simulink model "LIMP"  (R2014b)
settings: Solver=ode3  StartTime=0.0  StopTime=10.0  FixedStep=0.01  RelTol=1e-3
values from neighbouring files (symbols this model uses):
  G = 9.81    [main.m]
  i = max(find(p > availablepercentiles))    [cmaes.m]
  x = 100 * (x.^2 - y) + (x - 1).^2    [cmaes.m]    (also in ddp_naive.m = zeros(nx, n+1); main.m = 0; p1_plan001.mat = [0 2.16226505425e-05 9.59496359766e-05 0.00022595251555 0.00; p1_sim.m = S(:, 1))
  xd = 0    [main.m]    (also in p1_plan001.mat = [0 0.000462576080308 0.00102632112351 0.0015734075806 0.0021; p1_sim.m = S(:, 3); processData.m = Sxd.Data(end))
  y = repmat(scale, 1, size(x,2)) .* x    [cmaes.m]    (also in main.m = 0; p1_plan001.mat = [0 -1.26027772298e-05 -5.49591014786e-05 -0.00012654563427 -; p1_sim.m = S(:, 2); p2_ddp_run.m = vars.y)
  yd = 0    [main.m]    (also in p1_plan001.mat = [0 -0.000268095565629 -0.000576196670308 -0.000853920776779 ; p1_sim.m = S(:, 4); processData.m = Syd.Data(end))
  z = 1    [main.m]
undefined symbols (not defined in the file or in its folder): limp
libraries: simulink x1
settings Model: Creator=tianyuchen  LastModifiedBy=tianyuchen

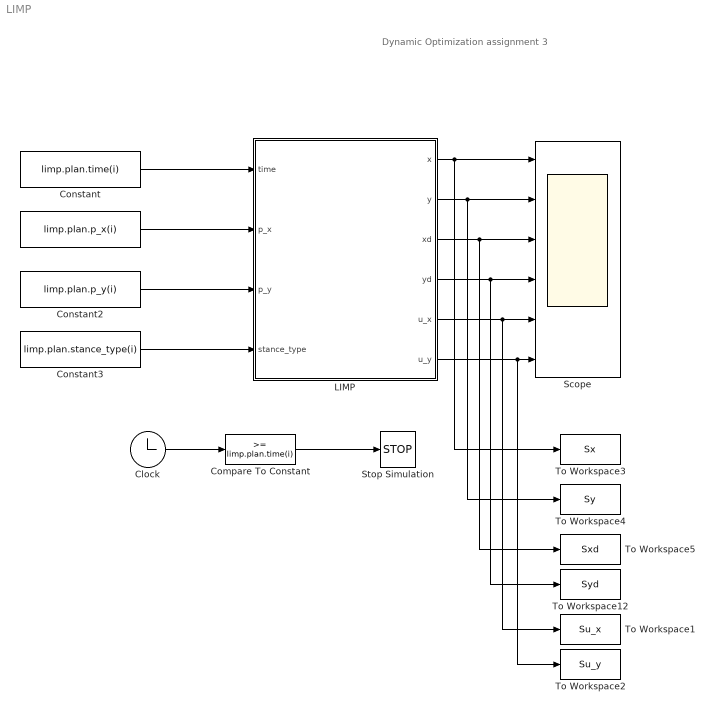
== system LIMP ==
  note: Dynamic Optimization
      | assignment 3
  " " : Constant  Value=limp.plan.p_x(i)
  Clock : Clock
  Compare To Constant : simulink/Logic and Bit Operations/Compare To Constant  relop=>=  const=limp.plan.time(i)  OutDataTypeStr=boolean
  Constant : Constant  Value=limp.plan.time(i)
  Constant2 : Constant  Value=limp.plan.p_y(i)
  Constant3 : Constant  Value=limp.plan.stance_type(i)
  LIMP : Subsystem
  Scope : Scope  NumInputPorts=6
      settings: TickLabels=on  ShowLegends=on  YMin=-5~-5~-5~-5~-5~-5  YMax=5~5~5~5~5~5  ScrollMode=on
  Stop Simulation : Stop
  To Workspace1 : ToWorkspace  VariableName=Su_x  SaveFormat=Timeseries  SampleTime=-1
  To Workspace12 : ToWorkspace  VariableName=Syd  SaveFormat=Timeseries  SampleTime=-1
  To Workspace2 : ToWorkspace  VariableName=Su_y  SaveFormat=Timeseries  SampleTime=-1
  To Workspace3 : ToWorkspace  VariableName=Sx  SaveFormat=Timeseries  SampleTime=-1
  To Workspace4 : ToWorkspace  VariableName=Sy  SaveFormat=Timeseries  SampleTime=-1
  To Workspace5 : ToWorkspace  VariableName=Sxd  SaveFormat=Timeseries  SampleTime=-1
  wires:
  Constant/1 -> LIMP/1(time)
  " "/1 -> LIMP/2(p_x)
  Constant2/1 -> LIMP/3(p_y)
  Constant3/1 -> LIMP/4(stance_type)
  Clock/1 -> Compare To Constant/1
  Compare To Constant/1 -> Stop Simulation/1
  LIMP/2(y) -> To Workspace4/1, Scope/2
  LIMP/3(xd) -> To Workspace5/1, Scope/3
  LIMP/4(yd) -> To Workspace12/1, Scope/4
  LIMP/6(u_y) -> To Workspace2/1, Scope/6
  LIMP/5(u_x) -> To Workspace1/1, Scope/5
  LIMP/1(x) -> To Workspace3/1, Scope/1

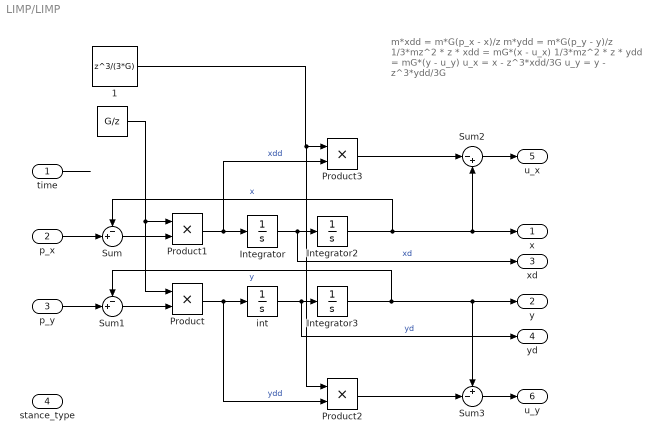
== system LIMP/LIMP ==
  note: m*xdd = m*G(p_x - x)/z
      | m*ydd = m*G(p_y - y)/z
      | 1/3*mz^2 * z * xdd = mG*(x - u_x)
      | 1/3*mz^2 * z * ydd = mG*(y - u_y)
      |
      | u_x = x - z^3*xdd/3G
      | u_y = y - z^3*ydd/3G
  time : Inport
  p_x : Inport  Port=2
  p_y : Inport  Port=3
  stance_type : Inport  Port=4
  " " : Constant  Value=G/z
  " 1" : Constant  Value=z^3/(3*G)
  Integrator : Integrator  InitialCondition=xd
  Integrator2 : Integrator  InitialCondition=x
  Integrator3 : Integrator  InitialCondition=y
  Product{,1..3} (4 alike) : Product
  Sum : Sum  Inputs=-+|
  Sum1 : Sum  Inputs=-+|
  Sum2 : Sum  Inputs=|-+
  Sum3 : Sum  Inputs=+-|
  int : Integrator  InitialCondition=yd
  x : Outport
  y : Outport  Port=2
  xd : Outport  Port=3
  yd : Outport  Port=4
  u_x : Outport  Port=5
  u_y : Outport  Port=6
  wires:
  time/1 -> ?
  " "/1 -> Product1/1, Product/1
  p_x/1 -> Sum/2
  Sum/1 -> Product1/2
  p_y/1 -> Sum1/2
  Sum1/1 -> Product/2
  Product1/1 -> Product3/2, Integrator/1  "xdd"
  Product/1 -> Product2/2, int/1  "ydd"
  Integrator/1 -> xd/1, Integrator2/1  "xd"
  int/1 -> yd/1, Integrator3/1  "yd"
  Integrator2/1 -> Sum/1, Sum2/2, x/1  "x"
  Integrator3/1 -> Sum3/1, y/1, Sum1/1  "y"
  Sum2/1 -> u_x/1
  Sum3/1 -> u_y/1
  " 1"/1 -> Product3/1, Product2/1
  Product3/1 -> Sum2/1
  Product2/1 -> Sum3/2
